simulink model "OSCILOS_Sim_nonlin"  (R2015a)
settings: Solver=ode3  StartTime=0.0  StopTime=1.5  FixedStep=dt  RelTol=1e-3
model workspace: external: MATLAB File /Users/amorgans/Documents/amorgans/OSCILOS/OSCILOS_SIM/parameters.m (data not in the file)
values from neighbouring files (symbols this model uses):
  dt = 10^-5    (= 1e-05)    [parameters.m]
libraries: OSCILOS_SIM x6
settings Model: CovSFcnEnable=off  Creator=Maxi  LastModifiedBy=amorgans
settings DebuggingCC: SolverPrmCheckMsg=warning

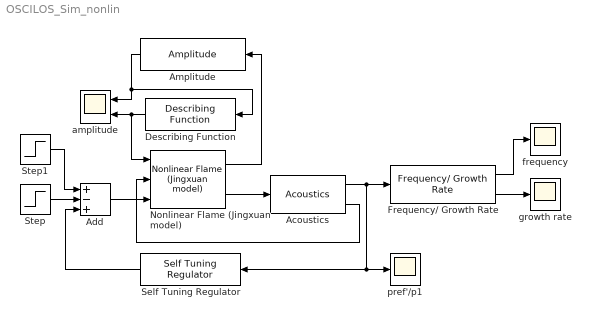
== system OSCILOS_Sim_nonlin ==
  Acoustics : OSCILOS_SIM/Acoustics  SystemSampleTime=-1
  Add : Sum  Inputs=+-+
  Amplitude : OSCILOS_SIM/Amplitude  SystemSampleTime=-1
  Describing Function : OSCILOS_SIM/Describing Function  SystemSampleTime=-1
  Frequency/ Growth Rate : OSCILOS_SIM/Frequency// Growth Rate  SystemSampleTime=-1
  Nonlinear Flame (Jingxuan model) : OSCILOS_SIM/Nonlinear Flame (Jingxuan model)  SystemSampleTime=-1
  "Self Tuning Regulator " : OSCILOS_SIM/Self Tuning Regulator   SystemSampleTime=-1
  Step : Step  Time=dt*2  SampleTime=0
  Step1 : Step  Time=0  SampleTime=0
  amplitude : Scope  NumInputPorts=2
      settings: YMin=-5~-5  YMax=5~5  SaveName=ScopeData4
  frequency : Scope
      settings: SaveName=ScopeData2
  growth rate : Scope
  pref'/p1 : Scope
      settings: TimeRange=1.5  YMin=3.372549019607844  YMax=4.972549019607844
  wires:
  Acoustics/2 -> Nonlinear Flame (Jingxuan model)/2
  Nonlinear Flame (Jingxuan model)/2 -> Acoustics/1
  Describing Function/1 -> amplitude/2, Nonlinear Flame (Jingxuan model)/1
  Acoustics/1 -> pref'/p1/1, "Self Tuning Regulator "/1, Frequency/ Growth Rate/1
  Add/1 -> Nonlinear Flame (Jingxuan model)/3
  "Self Tuning Regulator "/1 -> Add/3
  Step/1 -> Add/2
  Step1/1 -> Add/1
  Frequency/ Growth Rate/2 -> growth rate/1
  Frequency/ Growth Rate/1 -> frequency/1
  Amplitude/1 -> Describing Function/1, amplitude/1
  Nonlinear Flame (Jingxuan model)/1 -> Amplitude/1
